simulink model "altitude_from_pitch_loop"  (R2019a)
settings: Solver=VariableStepAuto  StartTime=0.0  StopTime=10000  RelTol=1e-3
values from neighbouring files (symbols this model uses):
  AP = 9.81    [wind_parameters.sldd]
undefined symbols (not defined in the file or in its folder): WIND
libraries: simulink x1
settings Model: Creator=nikhil  LastModifiedBy=VTOL_HYD

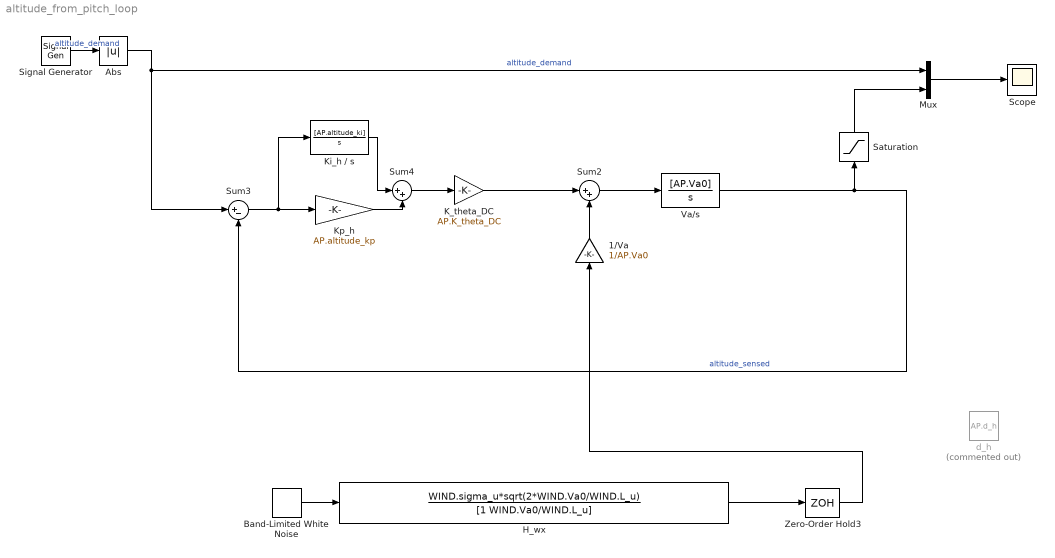
== system altitude_from_pitch_loop ==
  1/Va : Gain  Gain=1/AP.Va0
  Abs : Abs
  Band-Limited White Noise : simulink/Sources/Band-Limited White Noise  Cov=[1]  Ts=0.001  seed=[23341]
  H_wx : TransferFcn  InitFcn=|  Numerator=WIND.sigma_u*sqrt(2*WIND.Va0/WIND.L_u)  Denominator=[1 WIND.Va0/WIND.L_u]
      | addpath('.')
      | wind_parameters
      | simulation_parameters
  K_theta_DC : Gain  Gain=AP.K_theta_DC
  Ki_h / s : TransferFcn  Numerator=[AP.altitude_ki]  Denominator=[1 0]
  Kp_h : Gain  Gain=AP.altitude_kp
  Mux : Mux  Inputs=2
  Saturation : Saturate  UpperLimit=10000
  Scope : Scope
  Signal Generator : SignalGenerator  Amplitude=100  Frequency=50  Units=rad/sec
  Sum2 : Sum  Inputs=|++
  Sum3 : Sum  Inputs=|+-
  Sum4 : Sum  Inputs=|++
  Va/s : TransferFcn  Numerator=[AP.Va0]  Denominator=[1 0]
  Zero-Order Hold3 : ZeroOrderHold  SampleTime=-1
  d_h : Constant  Commented=on  Value=AP.d_h
  wires:
  Va/s/1 -> Sum3/2, Saturation/1  "altitude_sensed"
  Mux/1 -> Scope/1
  Sum4/1 -> K_theta_DC/1
  Ki_h / s/1 -> Sum4/1
  Kp_h/1 -> Sum4/2
  Abs/1 -> Sum3/1, Mux/1  "altitude_demand"
  Sum3/1 -> Ki_h / s/1, Kp_h/1
  1/Va/1 -> Sum2/2
  Zero-Order Hold3/1 -> 1/Va/1
  Sum2/1 -> Va/s/1
  Saturation/1 -> Mux/2
  K_theta_DC/1 -> Sum2/1
  Signal Generator/1 -> Abs/1  "altitude_demand"
  H_wx/1 -> Zero-Order Hold3/1
  Band-Limited White Noise/1 -> H_wx/1
